simulink model "HeartPacemakerModel"  (R2018a)
settings: Solver=VariableStepAuto  StartTime=0.0  StopTime=50  RelTol=1e-3
undefined symbols (not defined in the file): ecgVals, ecgValsSlow
settings Model: PauseTimes=.1  NumberOfSteps=10  Creator=root  LastModifiedBy=banks
settings CodeAppCC: StateflowObjectComments=on

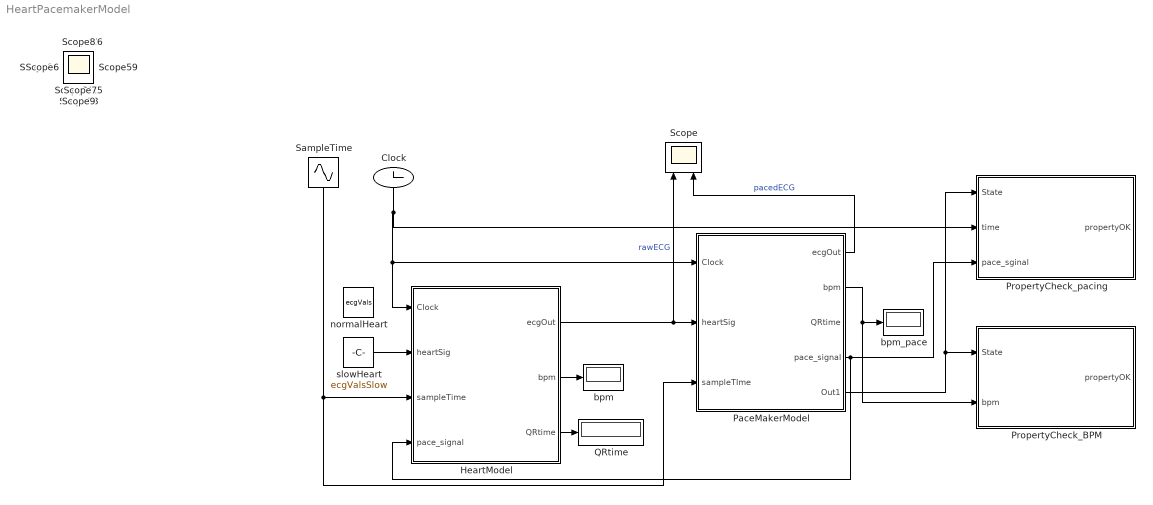
== system HeartPacemakerModel ==
  Clock : Clock
  HeartModel : Subsystem
  PaceMakerModel : Subsystem
  PropertyCheck_BPM : Stateflow chart  TreatAsAtomicUnit=on
  PropertyCheck_pacing : Stateflow chart  TreatAsAtomicUnit=on
  QRtime : Display
  SampleTime : Sin  Frequency=1000  SampleTime=0
  Scope : Scope  NumInputPorts=2
      settings: Tag=ECG
  bpm : Display
  bpm_pace : Display
  normalHeart : Constant  Value=ecgVals
  slowHeart : Constant  Value=ecgValsSlow
  Scope{1..12,14..16,18..19,21} (18 alike) : Scope
  wires:
  HeartModel/1(ecgOut) -> PaceMakerModel/2(heartSig), Scope/1  "rawECG"
  HeartModel/2(bpm) -> bpm/1
  HeartModel/3(QRtime) -> QRtime/1
  Clock/1 -> PaceMakerModel/1(Clock), HeartModel/1(Clock), PropertyCheck_pacing/2(time)
  PaceMakerModel/1(ecgOut) -> Scope/2  "pacedECG"
  SampleTime/1 -> HeartModel/3(sampleTime), PaceMakerModel/3(sampleTIme)
  PaceMakerModel/5(Out1) -> PropertyCheck_pacing/1(State), PropertyCheck_BPM/1(State)
  PaceMakerModel/2(bpm) -> PropertyCheck_BPM/2(bpm), bpm_pace/1
  PaceMakerModel/4(pace_signal) -> PropertyCheck_pacing/3(pace_sginal), HeartModel/4(pace_signal)
  slowHeart/1 -> HeartModel/2(heartSig)

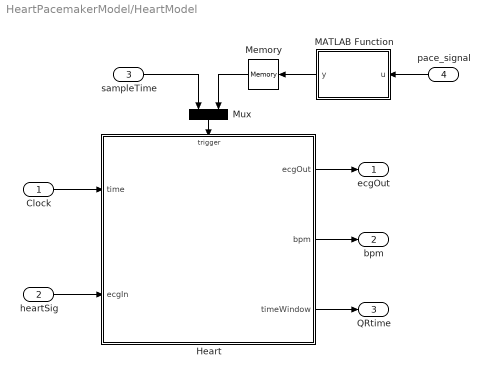
== system HeartPacemakerModel/HeartModel ==
  Clock : Inport
  heartSig : Inport  Port=2
  sampleTime : Inport  Port=3
  pace_signal : Inport  Port=4
  Heart : Stateflow chart  TreatAsAtomicUnit=on
  MATLAB Function : MATLAB Function  TreatAsAtomicUnit=on
  Memory : Memory
  Mux : Mux  Inputs=2
  ecgOut : Outport
  bpm : Outport  Port=2
  QRtime : Outport  Port=3
  wires:
  Heart/1(ecgOut) -> ecgOut/1
  Clock/1 -> Heart/1(time)
  sampleTime/1 -> Mux/1
  Heart/2(bpm) -> bpm/1
  heartSig/1 -> Heart/2(ecgIn)
  Heart/3(timeWindow) -> QRtime/1
  Mux/1 -> Heart/Trigger
  pace_signal/1 -> MATLAB Function/1(u)
  Memory/1 -> Mux/2
  MATLAB Function/1(y) -> Memory/1

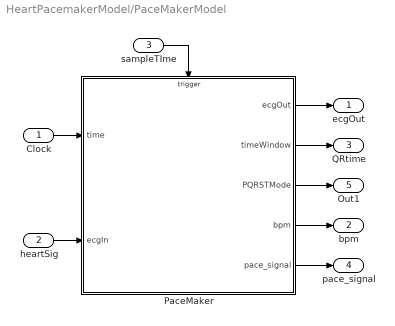
== system HeartPacemakerModel/PaceMakerModel ==
  Clock : Inport
  heartSig : Inport  Port=2
  sampleTIme : Inport  Port=3
  PaceMaker : Stateflow chart  TreatAsAtomicUnit=on
  ecgOut : Outport
  bpm : Outport  Port=2
  QRtime : Outport  Port=3
  pace_signal : Outport  Port=4
  Out1 : Outport  Port=5
  wires:
  PaceMaker/3(" PQRSTMode") -> Out1/1
  PaceMaker/1(ecgOut) -> ecgOut/1
  sampleTIme/1 -> PaceMaker/Trigger
  heartSig/1 -> PaceMaker/2(ecgIn)
  PaceMaker/2(timeWindow) -> QRtime/1
  PaceMaker/5(pace_signal) -> pace_signal/1
  Clock/1 -> PaceMaker/1(time)
  PaceMaker/4(bpm) -> bpm/1

== stateflow chart HeartPacemakerModel/PropertyCheck_pacing ==
  state Initial_State
  state Property
    state Initial_State
      en:
      propertyOK = 1,
      error_event = 0,
      t2 = time;
    state Pace
    state Error_State
      en:
      error_event = 1
    (default) -> Property.Initial_State
    Property.Initial_State -> Pace : [time - t2 > .115]
    Pace -> Property.Error_State : [State == 3 && pace_sginal == 0]
        | {propertyOK = 0}
  state Error_State
  (default) -> Initial_State
  Initial_State -> Property : [State == 2]
  Property -> Initial_State [order 2] : [State == 3 & propertyOK == 1]
  Property -> Error_State [order 3] : [error_event==1]
  Property -> Error_State [order 4] : [propertyOK == 0]
  Property -> Error_State [order 1] : [State == 3 & ...
      | propertyOK == 0]
  data: State input; error_event local; propertyOK output; time input; t2 local; pace_sginal input

== matlab function HeartPacemakerModel/HeartModel/MATLAB Function ==
  data: u input boolean; y output double
function y = fcn(u)
    if islogical(u)
        y = double(u);
    else
        y = 0.0;
    end
  

end

== stateflow chart HeartPacemakerModel/HeartModel/Heart ==
  settings: executeAtInitialization=1
  state HeartModel
    en:
    i=1;
    paceReceived = 0;
    state PQRST [parallel]
      en, du: ecgOut = sigVal;
      settings: executionOrder=1
      state impulse
        en: while(ecgIn(i) ~= -.14)
        send(advance, HeartModel.timer)
        end
        ex:paceReceived = 0;
      state reset
        en:
        beats = beats +1;
      state P
        en:t2 = time;
      state Q
        en:timeWindow = time-t2;
      state R
      state Rpeak
      state T
      state S
      P -> impulse [order 1] : [time - t2 > .11 && paceReceived]
      (default) -> reset
      impulse -> Q
      P -> Q [order 2] : [sigVal < -.09]
      reset -> P : [sigVal > .16]
      Q -> R : [sigVal >=.6]
      T -> reset : [sigVal < .04]{bpm = beats / time * 60}
      R -> Rpeak : [sigVal >=.6]
      S -> T : [sigVal > .2]
      Rpeak -> S : [sigVal < -.1]
    state sigWatcher [parallel]
      settings: executionOrder=3
      state check
        ex:paceReceived = 1;
      state sigRcvd
      (default) -> check
      check -> sigRcvd : [pace_signal]
      sigRcvd -> check : [paceReceived == 0]
    state timer [parallel]
      settings: executionOrder=2
      state a
        en:sigVal = ecgIn(i);
        t1= time;
        i = i + 1;
        if(i == length(ecgIn + 1))
        i = 1;
        end
      (default) -> a
      a -> a [order 2] : [advance]
      a -> a [order 1] : [time-t1 >=.025]
  data: ecgOut output double =0; time input; t1 local; ecgIn input; sigVal local =0; i local; bpm output =0; beats local =0; timeWindow output; t2 local; paceReceived local
  events: sample_rate input RISING_EDGE_EVENT; advance local FUNCTION_CALL_EVENT; pace_signal input RISING_EDGE_EVENT

== stateflow chart HeartPacemakerModel/PaceMakerModel/PaceMaker ==
  settings: executeAtInitialization=1
  state PaceModel
    en:
    state sigWatcher [parallel]
      settings: executionOrder=2
      state a
        en,du: sigVal = ecgIn;
      (default) -> a
    state PQRST [parallel]
      en, du: ecgOut = sigVal;
      settings: executionOrder=1
      state impulse
        en:send(pace_signal);
        while(ecgIn ~= -.14)
        end
      state reset
        ex:
        beats = beats+1
      state P
        en:t2 = time;
      state Q
        en:timeWindow = time-t2;
      state R
      state Rpeak
      state T
      state S
      P -> impulse [order 2] : [time - t2 > .115]
      (default) -> reset
      impulse -> Q
      P -> Q [order 1] : [sigVal < -.09]
      reset -> P : [sigVal > .16]
      Q -> R : [sigVal >=.6]
      T -> reset : [sigVal < .04]{bpm = beats / time * 60}
      R -> Rpeak : [sigVal >=.6]
      S -> T : [sigVal > .2]
      Rpeak -> S : [sigVal < -.1]
  data: ecgOut output double =0; time input; ecgIn input; sigVal local =0; timeWindow output; t2 local; PQRSTMode output Enum: PQRSTModeType; bpm output =0; beats local =0
  events: sample_rate input RISING_EDGE_EVENT; pace_signal output EITHER_EDGE_EVENT

== stateflow chart HeartPacemakerModel/PropertyCheck_BPM ==
  state Initial_State
  state Error_State
  state Pattern
    state Initial_State
      en:
      error_event = 0,
      propertyOK = 1;
    state Error_State
      en:
      error_event = 1
    (default) -> Pattern.Initial_State
    Pattern.Initial_State -> Pattern.Error_State : [State == 1 & bpm > 68]
        | {propertyOK = 0}
  (default) -> Initial_State
  Initial_State -> Pattern : [State == 7]
  Pattern -> Initial_State [order 2] : [State == 1 ...
      | & propertyOK == 1]
  Pattern -> Error_State [order 1] : [error_event == 1]
  Pattern -> Error_State [order 3] : [propertyOK == 0]
  data: State input; bpm input; error_event local; propertyOK output
